simulink model "LinearActuator"  (R2015a)
settings: Solver=ode45  StartTime=0.0  StopTime=10.0  MaxStep=0.1  RelTol=1e-3
undefined symbols (not defined in the file): Ta
settings Model: FPTRunName=Active  ModifiedByFormat=The MathWorks Inc.  CovSFcnEnable=off  Creator=The MathWorks Inc.  LastModifiedBy=The MathWorks Inc.
settings ConfigSet: ConfigType=Model
settings SolverCC: Priority=auto
settings DataIOCC: SaveOutput=off  SaveTime=off  SignalLoggingName=LinearActuator
settings OptimizationCC: InlineParamsCompatibleMode=off  ExpressionDepthLimit=2147483647  InitFltsAndDblsToZero=on  ForceBlockIOInitOptimize=off  EvaledLifeSpan=1  SimCompilerOptimization=Off
settings DebuggingCC: SaveWithParameterizedLinksMsg=none  UnderspecifiedInitializationDetection=Classic  MergeDetectMultiDrivingBlocksExec=none  SignalResolutionControl=TryResolveAllWithWarning  SolverPrmCheckMsg=warning  MultiTaskDSMMsg=warning  MultiTaskCondExecSysMsg=none  FcnCallInpInsideContextMsg=UseLocalSettings  AllowSymbolicDim=off  StateNameClashWarn=warning  SFMismatchInSimAndRtwBecauseOfMissingDataTypeDiag=warning
settings ModelReferenceCC: ModelReferenceMinAlgLoopOccurrences=on
settings RTWCC: EnableTagging=off  RTWCompilerOptimization=Off
settings CodeAppCC: ParameterTuningSideEffectCode=Output function  AllmanStyle=off
settings GRTTargetCC: TargetFcnLib=ansi_tfl_tmw.mat  CombineOutputUpdateFcns=off  EnableShiftOperators=off  PortableWordSizesTransition=off  GenerateErtSFunctionTransition=off  CreateSILPILBlockTransition=None  CodeProfilingSaveOptionsTransition=SummaryOnly  CodeExecutionProfilingTransition=off  CodeProfilingInstrumentationTransition=off  CodeExecutionProfileVariableTransition=executionProfile  GRTInterface=on

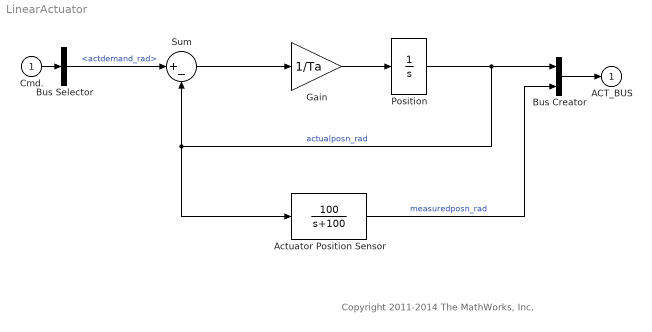
== system LinearActuator ==
  note: Copyright 2011-2014 The MathWorks, Inc.
  Cmd. : Inport  IOType=none  Commented=off  StatePerturbationForJacobian=1.0e-05  OutDataTypeStr=Bus: CONTROL_BUS
  Actuator Position Sensor : TransferFcn  IOType=none  Commented=off  StatePerturbationForJacobian=1.0e-05  Numerator=[100]  Denominator=[1 100]
  Bus Creator : BusCreator  IOType=none  Commented=off  StatePerturbationForJacobian=1.0e-05  Inputs=2  OutDataTypeStr=Bus: ACT_BUS
  Bus Selector : BusSelector  IOType=none  Commented=off  StatePerturbationForJacobian=1.0e-05  OutputSignals=actdemand_rad
  Gain : Gain  IOType=none  Commented=off  StatePerturbationForJacobian=1.0e-05  Gain=1/Ta  SaturateOnIntegerOverflow=on  OutDataTypeStr=Inherit: Same as input  ParamDataTypeStr=Inherit: Same as input
  Position : Integrator  IOType=none  Commented=off  StatePerturbationForJacobian=1.0e-05  UpperSaturationLimit=pi*45/180  LowerSaturationLimit=-pi*45/180
  Sum : Sum  IOType=none  Commented=off  StatePerturbationForJacobian=1.0e-05  Inputs=|+-  SaturateOnIntegerOverflow=on  InputSameDT=on  OutDataTypeStr=Inherit: Same as first input
  ACT_BUS : Outport  IOType=none  Commented=off  StatePerturbationForJacobian=1.0e-05  OutDataTypeStr=Bus: ACT_BUS  InitialOutput=0  BusOutputAsStruct=on
  wires:
  Actuator Position Sensor/1 -> Bus Creator/2  "measuredposn_rad"
  Position/1 -> Bus Creator/1, Actuator Position Sensor/1, Sum/2  "actualposn_rad"
  Gain/1 -> Position/1
  Sum/1 -> Gain/1
  Cmd./1 -> Bus Selector/1
  Bus Selector/1 -> Sum/1  "<actdemand_rad>"
  Bus Creator/1 -> ACT_BUS/1
